simulink model "franken_pp"  (R2021a)
settings: Solver=FixedStepAuto  StartTime=0.0  StopTime=10  FixedStep=Ts  RelTol=1e-3
values from neighbouring files (symbols this model uses):
  alpha = 0.55    [params.m]
  Be = 0    [params.m]
  beta = 0.25    [params.m]
  Bh = 20    [params.m]
  Bm = 50    [params.m]
  Bs = 50    [params.m]
  delay = 1    [params.m]
  Dh = 10    [params.m]
  Dm = 0    [params.m]
  Ds = 0    [params.m]
  Fip = 1    [params.m]
  H_d = 1    [params.m]
  Je = 0    [params.m]
  Jh = 0.5    [params.m]
  Ke = 20    [params.m]
  Kh = 50    [params.m]
  Km = 100    [params.m]
  Ks = 100    [params.m]
  Mm = 0.5    [params.m]
  Ms = 2    [params.m]
  Ph = 25    [params.m]
  Ts = 0.001    [params.m]
undefined symbols (not defined in the file or in its folder): tau
libraries: simulink x5
settings Model: PauseTimes=40  Creator=antoninoparisi  LastModifiedBy=antoninoparisi

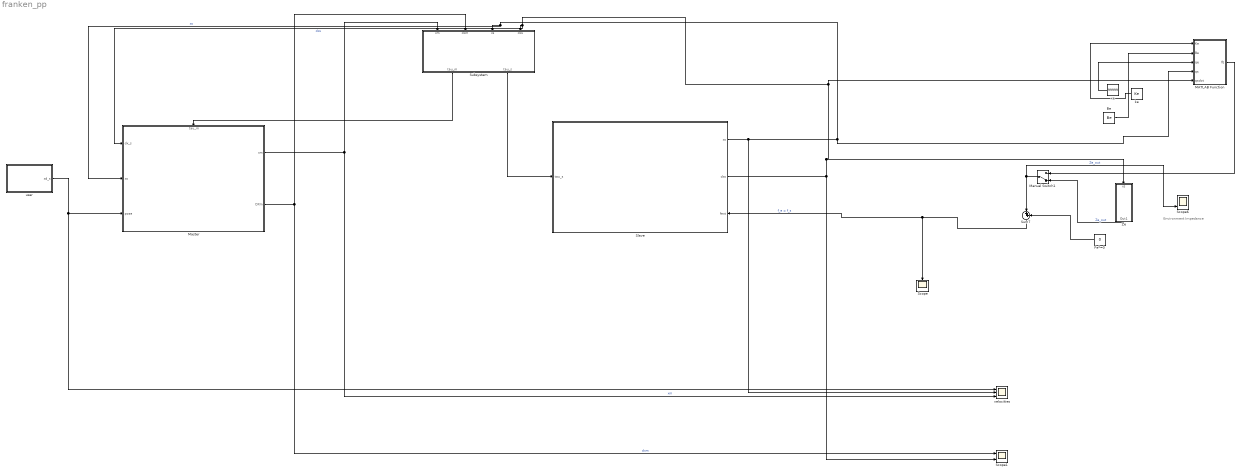
== system franken_pp ==
  note: Environment Impedance
  Be : Constant  Value=Be
  Fe*=0 : Constant  Value=0
  MATLAB Function : MATLAB Function  TreatAsAtomicUnit=on
  Manual Switch1 : ManualSwitch  CurrentSetting=0
  Master : Subsystem
      settings: PortSchema="{\"entries\":[{\"content\":{\"sides\":[{\"content\":{\"connectorIds\":[\"In1\",\"In2\",\"In3\"]},\"type\":\"ConnectorPlacement.EquallySpacedRectSide\",\"uuid\":\"1611af17-d019-4ea0-b30f-82f2e4a8e750\"},{\"content\":{\"connectorIds\":[\"Out1\",\"Out2\"],\"side\":\"RIGHT\"},\"type\":\"ConnectorPlacement.EquallySpacedRectSide\",\"uuid\":\"216ac5d0-4324-4f7d-99ca-2c077bed0ff3\"},{\"content\":{\"connectorIds\":[\"In4\"],\"side\":\"TOP\"},\"type\":\"ConnectorPlacement.EquallySpacedRectSide\",\"uuid\":\"270bcd60-bcfb-44eb-9993-004924a85997\"}]},\"type\":\"ConnectorPlacement.EquallySpacedConnector\",\"uuid\":\"754685d8-e0f3-4ed9-824d-c363b420fcd1\"}],\"packageUris\":[\"http://schema.mathworks.com/mf0/Connector/R2020b\"],\"version\":\"1.0\"}"
  Scope : Scope
  Scope1 : Scope  NumInputPorts=2
  Scope6 : Scope  NumInputPorts=2
  Slave : Subsystem
      settings: PortSchema="{\"entries\":[{\"content\":{\"sides\":[{\"content\":{\"connectorIds\":[\"In1\"]},\"type\":\"ConnectorPlacement.EquallySpacedRectSide\",\"uuid\":\"78b98c26-b3b3-4c1c-a2a9-2b1f81ca7a96\"},{\"content\":{\"connectorIds\":[\"Out1\",\"Out2\",\"In2\"],\"side\":\"RIGHT\"},\"type\":\"ConnectorPlacement.EquallySpacedRectSide\",\"uuid\":\"d1781ab8-1e84-4ce0-bcac-f4a6da9bce42\"},{\"content\":{\"connectorIds\":[],\"side\":\"TOP\"},\"type\":\"ConnectorPlacement.EquallySpacedRectSide\",\"uuid\":\"3a0b4df9-93f8-49a3-a565-44089873a5ef\"}]},\"type\":\"ConnectorPlacement.EquallySpacedConnector\",\"uuid\":\"1fdb1ec6-45bb-453f-97e9-2c7f461a82a3\"}],\"packageUris\":[\"http://schema.mathworks.com/mf0/Connector/R2020b\"],\"version\":\"1.0\"}"
  Subsystem : Subsystem
  Sum7 : Sum  Inputs=|++
  Ze : Subsystem
  ke : Constant  Value=Ke
  user : Subsystem
  velocities : Scope  NumInputPorts=3
  xe : Constant  Value=99999
  wires:
  Fe*=0/1 -> Sum7/2
  ke/1 -> MATLAB Function/1(Ke)
  xe/1 -> MATLAB Function/3(qe)
  Ze/1(Out1) -> Manual Switch1/2  "Ze_out"
  Be/1 -> MATLAB Function/2(Be)
  Manual Switch1/1 -> Sum7/1, Scope6/2  "Ze_out"
  MATLAB Function/1(fE) -> Manual Switch1/1
  user/1(xd_s) -> velocities/1, Master/3(pose)
  Slave/1(xs) -> velocities/2, MATLAB Function/4(qs), Master/2(xs), Subsystem/3(xs)  "xs"
  Sum7/1 -> Slave/2(fext), Scope/1  "f_e = f_s"
  Slave/2(dxs) -> Scope1/2, Ze/1(xs), Master/1(dx_s), Subsystem/4(dxs), MATLAB Function/5(qsdot)  "dxs"
  Subsystem/1(tau_m) -> Master/4(tau_m)
  Subsystem/2(tau_s) -> Slave/1(tau_s)
  Master/1(xm) -> velocities/3, Subsystem/1(xm)  "xm"
  Master/2(DXm) -> Scope1/1, Subsystem/2(dxm)  "dxm"

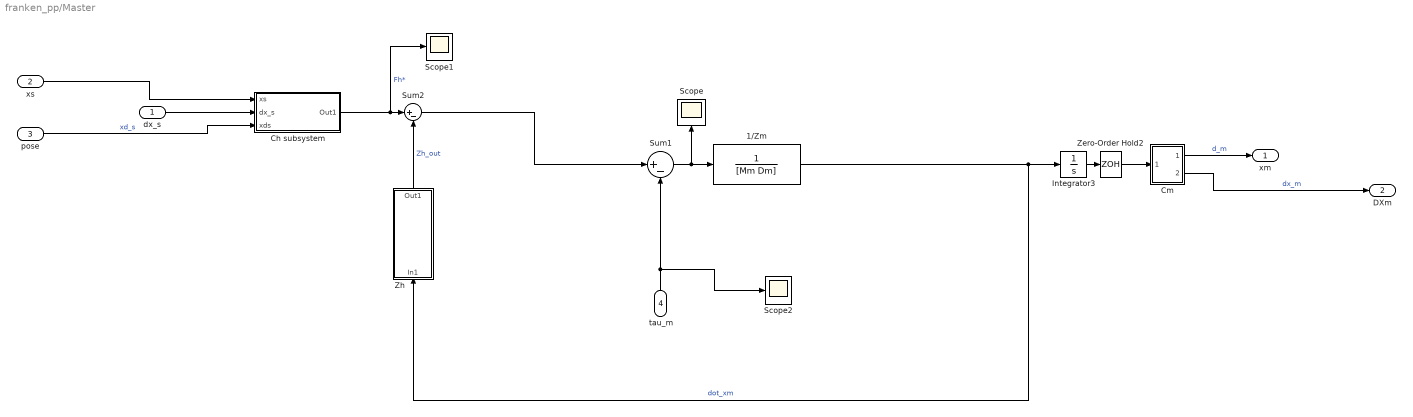
== system franken_pp/Master ==
  dx_s : Inport
  xs : Inport  Port=2
  pose : Inport  Port=3
  tau_m : Inport  Port=4
  1/Zm : TransferFcn  Denominator=[Mm Dm]
  Ch subsystem : Subsystem
  Cm : Subsystem
  Integrator3 : Integrator
  Scope : Scope
  Scope1 : Scope
  Scope2 : Scope
  Sum1 : Sum  Inputs=|+-
  Sum2 : Sum  Inputs=|+-
  Zero-Order Hold2 : ZeroOrderHold  SampleTime=-1
  Zh : Subsystem
  xm : Outport
  DXm : Outport  Port=2
  wires:
  Zh/1(Out1) -> Sum2/2  "Zh_out"
  1/Zm/1 -> Integrator3/1, Zh/1(In1)  "dot_xm"
  Zero-Order Hold2/1 -> Cm/1(In1)
  Integrator3/1 -> Zero-Order Hold2/1
  Ch subsystem/1(Out1) -> Scope1/1, Sum2/1  "Fh*"
  pose/1 -> Ch subsystem/3(xds)  "xd_s"
  xs/1 -> Ch subsystem/1(xs)
  Cm/2(DXm) -> DXm/1  "dx_m"
  dx_s/1 -> Ch subsystem/2(dx_s)
  Cm/1(Xm) -> xm/1  "d_m"
  Sum1/1 -> 1/Zm/1, Scope/1
  tau_m/1 -> Sum1/2, Scope2/1
  Sum2/1 -> Sum1/1

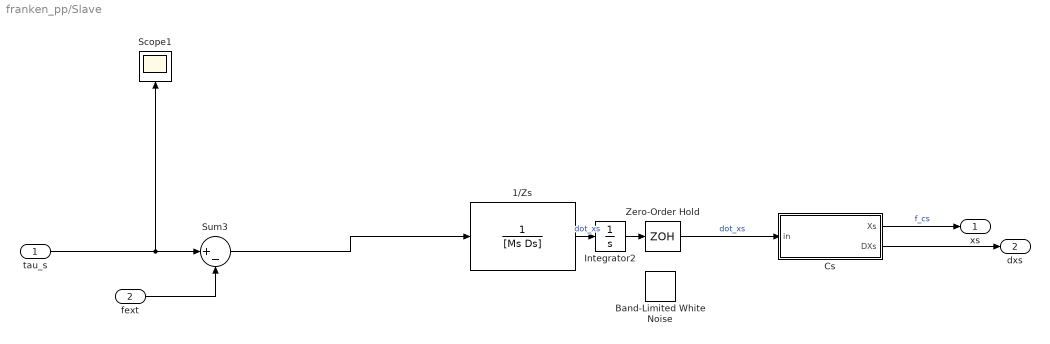
== system franken_pp/Slave ==
  tau_s : Inport
  fext : Inport  Port=2
  1/Zs : TransferFcn  Denominator=[Ms Ds]
  Band-Limited White Noise : simulink/Sources/Band-Limited White Noise  Cov=[0.000001]  Ts=Ts  seed=[23341]
  Cs : Subsystem
  Integrator2 : Integrator
  Scope1 : Scope
  Sum3 : Sum  Inputs=|+-
  Zero-Order Hold : ZeroOrderHold  SampleTime=-1
  xs : Outport
  dxs : Outport  Port=2
  wires:
  Zero-Order Hold/1 -> Cs/1(in)  "dot_xs"
  1/Zs/1 -> Integrator2/1  "dot_xs"
  Integrator2/1 -> Zero-Order Hold/1
  Cs/1(Xs) -> xs/1  "f_cs"
  Cs/2(DXs) -> dxs/1
  tau_s/1 -> Sum3/1, Scope1/1
  Sum3/1 -> 1/Zs/1
  fext/1 -> Sum3/2

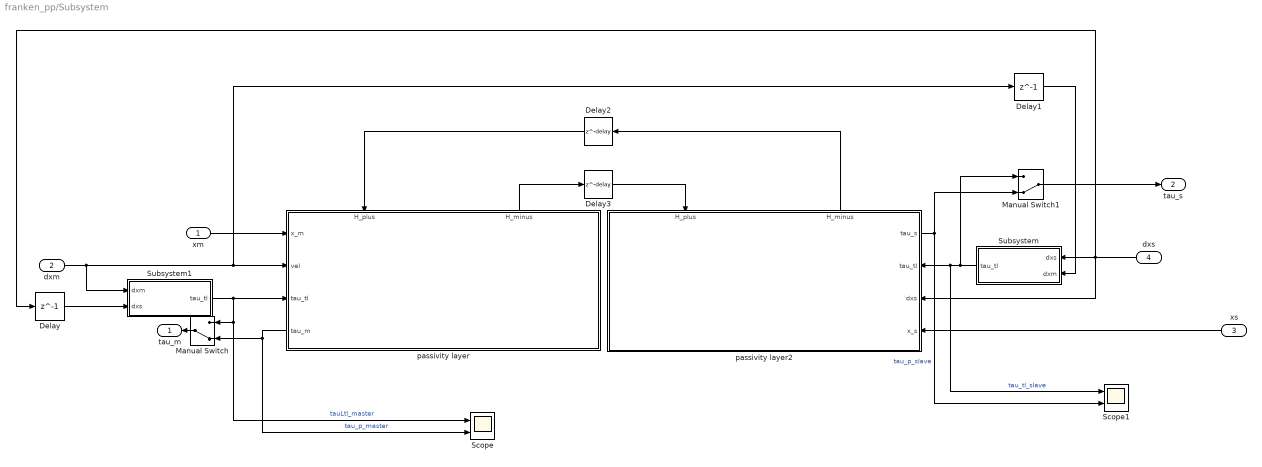
== system franken_pp/Subsystem ==
  xm : Inport
  dxm : Inport  Port=2
  xs : Inport  Port=3
  dxs : Inport  Port=4
  Delay : Delay  DelayLength=1  SampleTime=Ts
  Delay1 : Delay  DelayLength=1  SampleTime=Ts
  Delay2 : Delay  DelayLength=delay  SampleTime=Ts
  Delay3 : Delay  DelayLength=delay  SampleTime=Ts
  Manual Switch : ManualSwitch  CurrentSetting=0
  Manual Switch1 : ManualSwitch  CurrentSetting=0
  Scope : Scope  NumInputPorts=2
  Scope1 : Scope  NumInputPorts=2
  Subsystem : Subsystem
  Subsystem1 : Subsystem
  passivity layer : Subsystem
      settings: PortSchema="{\"entries\":[{\"content\":{\"sides\":[{\"content\":{\"connectorIds\":[]},\"type\":\"ConnectorPlacement.EquallySpacedRectSide\",\"uuid\":\"37bc6a68-8a11-4e98-9ac3-187f52517b60\"},{\"content\":{\"connectorIds\":[\"In4\",\"Out1\"],\"side\":\"RIGHT\"},\"type\":\"ConnectorPlacement.EquallySpacedRectSide\",\"uuid\":\"8a8e0676-f09b-4900-bb42-b008c53363bc\"},{\"content\":{\"connectorIds\":[\"Out2\",\"In1\",\"In2\",\"In3\"],\"side\":\"TOP\"},\"type\":\"ConnectorPlacement.EquallySpacedRectSide\",\"uuid\":\"476ab686-2607-4be6-9f50-5e1462be9089\"},{\"content\":{\"connectorIds\":[],\"side\":\"BOTTOM\"},\"type\":\"ConnectorPlacement.EquallySpacedRectSide\",\"uuid\":\"05cf8dac-5a1d-4d4a-b791-ec6ccb869d40\"}]},\"type\":\"ConnectorPlacement.EquallySpacedConnector\",\"uuid\":\"6a676768-9b76-4392-9dc3-eaadf2de8607\"}],\"packageUris\":[\"http://schema.mathworks.com/mf0/Connector/R2020b\"],\"version\":\"1.0\"}"
  passivity layer2 : Subsystem
      settings: PortSchema="{\"entries\":[{\"content\":{\"sides\":[{\"content\":{\"connectorIds\":[]},\"type\":\"ConnectorPlacement.EquallySpacedRectSide\",\"uuid\":\"37bc6a68-8a11-4e98-9ac3-187f52517b60\"},{\"content\":{\"connectorIds\":[\"In4\",\"Out1\"],\"side\":\"RIGHT\"},\"type\":\"ConnectorPlacement.EquallySpacedRectSide\",\"uuid\":\"8a8e0676-f09b-4900-bb42-b008c53363bc\"},{\"content\":{\"connectorIds\":[],\"side\":\"TOP\"},\"type\":\"ConnectorPlacement.EquallySpacedRectSide\",\"uuid\":\"476ab686-2607-4be6-9f50-5e1462be9089\"},{\"content\":{\"connectorIds\":[\"In1\",\"In2\",\"In3\",\"Out2\"],\"side\":\"BOTTOM\"},\"type\":\"ConnectorPlacement.EquallySpacedRectSide\",\"uuid\":\"05cf8dac-5a1d-4d4a-b791-ec6ccb869d40\"}]},\"type\":\"ConnectorPlacement.EquallySpacedConnector\",\"uuid\":\"6a676768-9b76-4392-9dc3-eaadf2de8607\"}],\"packageUris\":[\"http://schema.mathworks.com/mf0/Connector/R2020b\"],\"version\":\"1.0\"}"
  tau_m : Outport
  tau_s : Outport  Port=2
  wires:
  passivity layer/2(tau_m) -> Manual Switch/2, Scope/2  "tau_p_master"
  passivity layer2/2(tau_s) -> Scope1/2, Manual Switch1/2  "tau_p_slave"
  xm/1 -> passivity layer/3(x_m)
  dxm/1 -> Subsystem1/1(dxm), passivity layer/2(vel), Delay1/1
  Subsystem1/1(tau_tl) -> Scope/1, Manual Switch/1, passivity layer/1(tau_tl)  "tauLtl_master"
  Subsystem/1(tau_tl) -> Manual Switch1/1, Scope1/1, passivity layer2/3(tau_tl)  "tau_tl_slave"
  xs/1 -> passivity layer2/1(x_s)
  dxs/1 -> Delay/1, passivity layer2/2(dxs), Subsystem/1(dxs)
  Delay/1 -> Subsystem1/2(dxs)
  Delay1/1 -> Subsystem/2(dxm)
  passivity layer/1(H_minus) -> Delay3/1
  Delay3/1 -> passivity layer2/4(H_plus)
  Delay2/1 -> passivity layer/4(H_plus)
  passivity layer2/1(H_minus) -> Delay2/1
  Manual Switch/1 -> tau_m/1
  Manual Switch1/1 -> tau_s/1

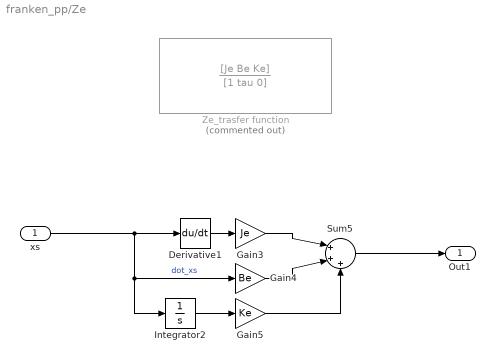
== system franken_pp/Ze ==
  xs : Inport
  Derivative1 : Derivative
  Gain3 : Gain  Gain=Je
  Gain4 : Gain  Gain=Be
  Gain5 : Gain  Gain=Ke
  Integrator2 : Integrator
  Sum5 : Sum  Inputs=|+++
  Ze_trasfer function : TransferFcn  Commented=on  Numerator=[Je Be Ke]  Denominator=[1 tau 0]
  Out1 : Outport
  wires:
  Gain4/1 -> Sum5/2
  Gain3/1 -> Sum5/1
  Gain5/1 -> Sum5/3
  Sum5/1 -> Out1/1
  Integrator2/1 -> Gain5/1
  xs/1 -> Integrator2/1, Gain4/1, Derivative1/1  "dot_xs"
  Derivative1/1 -> Gain3/1

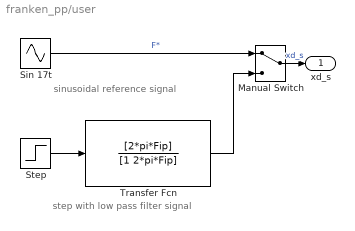
== system franken_pp/user ==
  note: step with low pass filter signal
  note: sinusoidal reference signal
  Manual Switch : ManualSwitch
  Sin 17t : Sin  Amplitude=0.5  Frequency=2*pi*0.5  SampleTime=Ts
  Step : Step  SampleTime=0
  Transfer Fcn : TransferFcn  Numerator=[2*pi*Fip]  Denominator=[1 2*pi*Fip]
  xd_s : Outport
  wires:
  Sin 17t/1 -> Manual Switch/1  "F*"
  Manual Switch/1 -> xd_s/1  "xd_s"
  Step/1 -> Transfer Fcn/1
  Transfer Fcn/1 -> Manual Switch/2

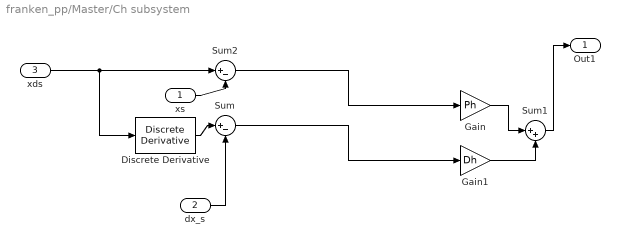
== system franken_pp/Master/Ch subsystem ==
  xs : Inport
  dx_s : Inport  Port=2
  xds : Inport  Port=3
  Discrete Derivative : simulink/Discrete/Discrete Derivative  gainval=1.0  ICPrevScaledInput=0.0  OutMin=[]  OutMax=[]  OutDataType=fixdt(1, 16)  OutScaling=2^-10  DoSatur=off
  Gain : Gain  Gain=Ph
  Gain1 : Gain  Gain=Dh
  Sum : Sum  Inputs=|+-
  Sum1 : Sum  Inputs=|++
  Sum2 : Sum  Inputs=|+-
  Out1 : Outport
  wires:
  Sum1/1 -> Out1/1
  Gain1/1 -> Sum1/2
  Gain/1 -> Sum1/1
  xs/1 -> Sum2/2
  Discrete Derivative/1 -> Sum/1
  Sum/1 -> Gain1/1
  Sum2/1 -> Gain/1
  xds/1 -> Sum2/1, Discrete Derivative/1
  dx_s/1 -> Sum/2

== system franken_pp/Master/Cm ==
  In1 : Inport
  Band-Limited White Noise : simulink/Sources/Band-Limited White Noise  Cov=[0.0000001]  Ts=Ts  seed=[23341]
  Discrete Derivative : simulink/Discrete/Discrete Derivative  gainval=1.0  ICPrevScaledInput=0.0  OutMin=[]  OutMax=[]  OutDataType=fixdt(1, 16)  OutScaling=2^-10  DoSatur=off
  Xm : Outport
  DXm : Outport  Port=2
  wires:
  Discrete Derivative/1 -> DXm/1
  In1/1 -> Xm/1, Discrete Derivative/1

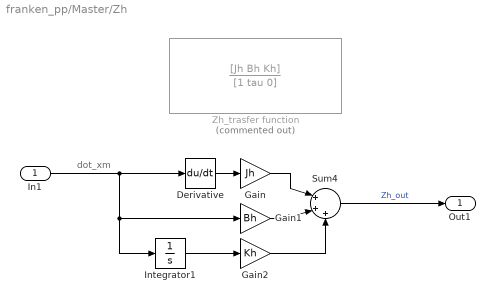
== system franken_pp/Master/Zh ==
  note: dot_xm
  In1 : Inport
  Derivative : Derivative
  Gain : Gain  Gain=Jh
  Gain1 : Gain  Gain=Bh
  Gain2 : Gain  Gain=Kh
  Integrator1 : Integrator
  Sum4 : Sum  Inputs=|+++
  Zh_trasfer function : TransferFcn  Commented=on  Numerator=[Jh Bh Kh]  Denominator=[1 tau 0]
  Out1 : Outport
  wires:
  Derivative/1 -> Gain/1
  Integrator1/1 -> Gain2/1
  Gain2/1 -> Sum4/3
  Gain1/1 -> Sum4/2
  Gain/1 -> Sum4/1
  Sum4/1 -> Out1/1  "Zh_out"
  In1/1 -> Gain1/1, Integrator1/1, Derivative/1

== system franken_pp/Slave/Cs ==
  in : Inport
  Discrete Derivative : simulink/Discrete/Discrete Derivative  gainval=1.0  ICPrevScaledInput=0.0  OutMin=[]  OutMax=[]  OutDataType=fixdt(1, 16)  OutScaling=2^-10  DoSatur=off
  Xs : Outport
  DXs : Outport  Port=2
  wires:
  in/1 -> Xs/1, Discrete Derivative/1
  Discrete Derivative/1 -> DXs/1

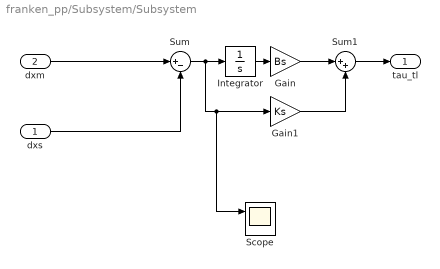
== system franken_pp/Subsystem/Subsystem ==
  dxs : Inport
  dxm : Inport  Port=2
  Gain : Gain  Gain=Bs
  Gain1 : Gain  Gain=Ks
  Integrator : Integrator
  Scope : Scope  NumInputPorts=2
  Sum : Sum  Inputs=|+-
  Sum1 : Sum  Inputs=|++
  tau_tl : Outport
  wires:
  dxm/1 -> Sum/1
  dxs/1 -> Sum/2
  Sum/1 -> Integrator/1, Scope/1, Gain1/1
  Integrator/1 -> Gain/1
  Gain/1 -> Sum1/1
  Gain1/1 -> Sum1/2
  Sum1/1 -> tau_tl/1

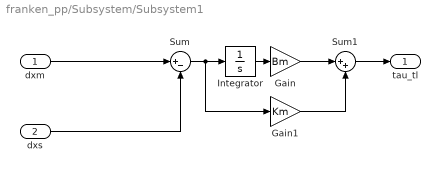
== system franken_pp/Subsystem/Subsystem1 ==
  dxm : Inport
  dxs : Inport  Port=2
  Gain : Gain  Gain=Bm
  Gain1 : Gain  Gain=Km
  Integrator : Integrator
  Sum : Sum  Inputs=|+-
  Sum1 : Sum  Inputs=|++
  tau_tl : Outport
  wires:
  dxm/1 -> Sum/1
  dxs/1 -> Sum/2
  Sum/1 -> Integrator/1, Gain1/1
  Integrator/1 -> Gain/1
  Gain/1 -> Sum1/1
  Gain1/1 -> Sum1/2
  Sum1/1 -> tau_tl/1

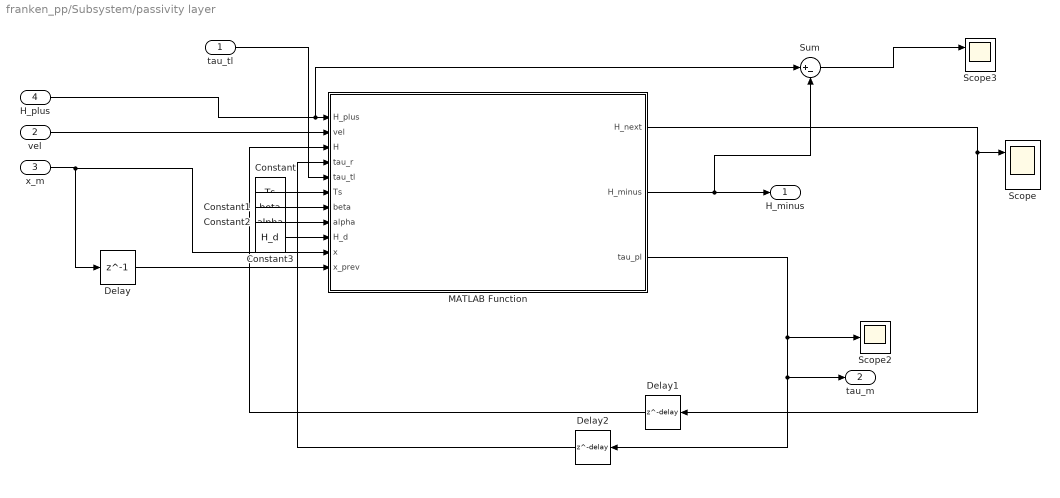
== system franken_pp/Subsystem/passivity layer ==
  tau_tl : Inport
  vel : Inport  Port=2
  x_m : Inport  Port=3
  H_plus : Inport  Port=4
  Constant : Constant  Value=Ts
  Constant1 : Constant  Value=beta
  Constant2 : Constant  Value=alpha
  Constant3 : Constant  Value=H_d
  Delay : Delay  DelayLength=1  SampleTime=Ts
  Delay1 : Delay  DelayLength=delay  InitialCondition=0  SampleTime=Ts
  Delay2 : Delay  DelayLength=delay  InitialCondition=0  SampleTime=Ts
  MATLAB Function : MATLAB Function  TreatAsAtomicUnit=on
  Scope : Scope  NumInputPorts=2
  Scope2 : Scope
  Scope3 : Scope  NumInputPorts=2
  Sum : Sum  Inputs=|+-
  H_minus : Outport
  tau_m : Outport  Port=2
  wires:
  MATLAB Function/1(H_next) -> Delay1/1, Scope/1
  MATLAB Function/2(H_minus) -> Sum/2, H_minus/1
  MATLAB Function/3(tau_pl) -> Delay2/1, tau_m/1, Scope2/1
  H_plus/1 -> Sum/1, MATLAB Function/1(H_plus)
  vel/1 -> MATLAB Function/2(vel)
  Delay1/1 -> MATLAB Function/3(H)
  x_m/1 -> MATLAB Function/10(x), Delay/1
  Delay/1 -> MATLAB Function/11(x_prev)
  Constant1/1 -> MATLAB Function/7(beta)
  Constant2/1 -> MATLAB Function/8(alpha)
  Constant3/1 -> MATLAB Function/9(H_d)
  Constant/1 -> MATLAB Function/6(Ts)
  Delay2/1 -> MATLAB Function/4(tau_r)
  tau_tl/1 -> MATLAB Function/5(tau_tl)
  Sum/1 -> Scope3/1

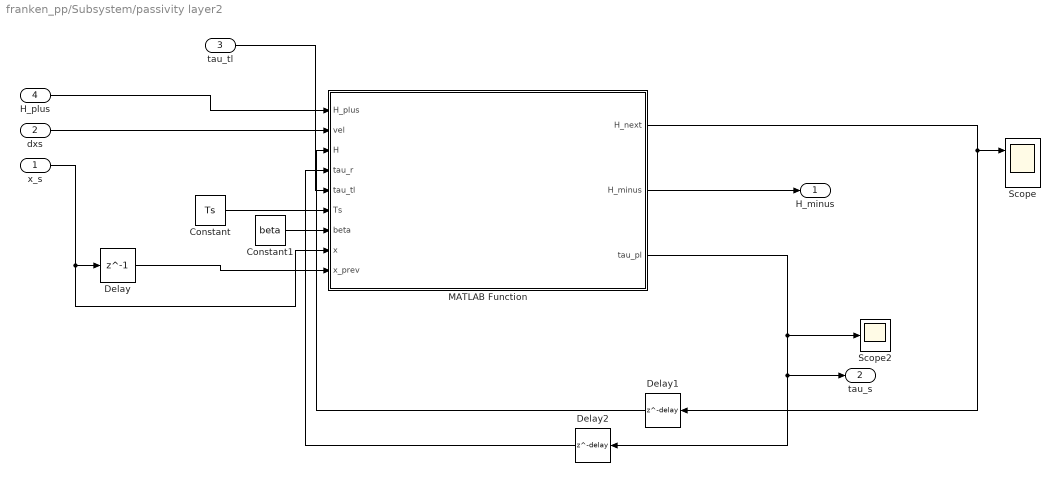
== system franken_pp/Subsystem/passivity layer2 ==
  x_s : Inport
  dxs : Inport  Port=2
  tau_tl : Inport  Port=3
  H_plus : Inport  Port=4
  Constant : Constant  Value=Ts
  Constant1 : Constant  Value=beta
  Delay : Delay  DelayLength=1  SampleTime=Ts
  Delay1 : Delay  DelayLength=delay  InitialCondition=0  SampleTime=Ts
  Delay2 : Delay  DelayLength=delay  InitialCondition=0  SampleTime=Ts
  MATLAB Function : MATLAB Function  TreatAsAtomicUnit=on
  Scope : Scope  NumInputPorts=2
  Scope2 : Scope
  H_minus : Outport
  tau_s : Outport  Port=2
  wires:
  MATLAB Function/1(H_next) -> Delay1/1, Scope/1
  MATLAB Function/2(H_minus) -> H_minus/1
  MATLAB Function/3(tau_pl) -> Delay2/1, tau_s/1, Scope2/1
  H_plus/1 -> MATLAB Function/1(H_plus)
  dxs/1 -> MATLAB Function/2(vel)
  Delay1/1 -> MATLAB Function/3(H)
  x_s/1 -> MATLAB Function/8(x), Delay/1
  Delay/1 -> MATLAB Function/9(x_prev)
  Constant1/1 -> MATLAB Function/7(beta)
  Constant/1 -> MATLAB Function/6(Ts)
  Delay2/1 -> MATLAB Function/4(tau_r)
  tau_tl/1 -> MATLAB Function/5(tau_tl)

== matlab function franken_pp/Subsystem/passivity layer2/MATLAB Function ==
  data: H_plus input; vel input; H input; tau_r input; H_next output; tau_tl input; H_minus output; tau_pl output; Ts input; beta input; x input; x_prev input
function [H_next,H_minus,tau_pl] = fcn(H_plus,vel,H,tau_r,tau_tl,Ts,beta,x,x_prev)



deltaH_i = tau_r * (x-x_prev);


H_actual = H + H_plus - deltaH_i;

H_minus = 0;

if(H_actual > 0)
H_minus =  beta*H_actual;
end

H_next = H_actual - H_minus;

tau_max_1 = tau_tl;
if(H_next <= 0)
    tau_max_1 = 0;
end



tau_max_2 = H_next/(vel*Ts);



tau_pl = sign(tau_tl)*min(abs([tau_tl,tau_max_1,tau_max_2])) ;

== matlab function franken_pp/MATLAB Function ==
  data: Ke input; fE output; Be input; qe input; qs input; qsdot input
function fE = environment(Ke, Be, qe, qs, qsdot)
    if qs > qe
        fE = Ke * (qs - qe) + Be * qsdot;
    else
        fE = 0;
    end
end

== matlab function franken_pp/Subsystem/passivity layer/MATLAB Function ==
  data: H_plus input; vel input; H input; tau_r input; H_next output; tau_tl input; H_minus output; tau_pl output; Ts input; beta input; alpha input; H_d input; x input; x_prev input
function [H_next,H_minus,tau_pl] = fcn(H_plus,vel,H,tau_r,tau_tl,Ts,beta,alpha,H_d,x,x_prev)


deltaH_i = tau_r * (x-x_prev);

H_actual = H + H_plus - deltaH_i;

H_minus = 0;


if(H_actual > 0)
H_minus =  beta*H_actual;
end

H_next = H_actual - H_minus;

tau_max_1 = tau_tl;

if(H_next <= 0)
    tau_max_1 = 0;
end

tau_max_2 = H_next/(vel*Ts);


if(H_d > H_next)
    tau_tlc = - alpha*(H_d - H_next) * vel;
else
    tau_tlc=0;   
end

% 
% if(H_actual > 2*H_d)
%     H_next = H_d;
% end
% 



tau_pl = sign(tau_tl)*min(abs([tau_tl,tau_max_1,tau_max_2])) + tau_tlc;
